simulink model "integrator_12B"  (Simulink 8.0)
settings: Solver=FixedStepDiscrete  StartTime=0.0  StopTime=10.0  FixedStep=1  RelTol=1e-3
libraries: simulink x1
settings Model: Creator=elliocm  LastModifiedBy=elliocm
settings DebuggingCC: IntegerOverflowMsg=none
settings CodeAppCC: CustomSymbolStrType=$N$R$M_T  InternalIdentifier=Shortened
settings ConfigComp: Description=Design Verifier Custom Configuration Component  DVMaxProcessTime=5000  DVMaxTestCaseSteps=500  DVTestSuiteOptimization=CombinedObjectives (Nonlinear Extended)

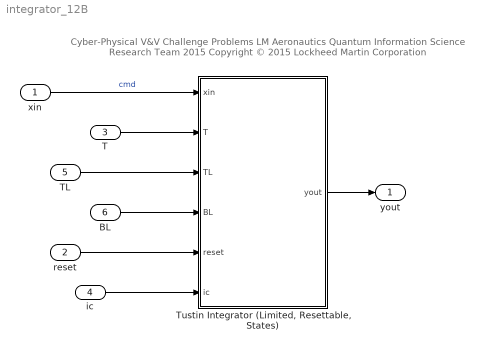
== system integrator_12B ==
  note: Cyber-Physical V&V Challenge Problems
      | LM Aeronautics Quantum Information Science Research Team 2015
      | Copyright © 2015 Lockheed Martin Corporation
  xin : Inport  OutDataTypeStr=double
  reset : Inport  Port=2  OutDataTypeStr=boolean
  T : Inport  Port=3  OutDataTypeStr=double
  ic : Inport  Port=4  OutDataTypeStr=double
  TL : Inport  Port=5  OutDataTypeStr=double
  BL : Inport  Port=6  OutDataTypeStr=double
  "Tustin Integrator (Limited, Resettable, States)" : Subsystem
  yout : Outport
  wires:
  BL/1 -> "Tustin Integrator (Limited, Resettable, States)"/4(BL)
  TL/1 -> "Tustin Integrator (Limited, Resettable, States)"/3(TL)
  reset/1 -> "Tustin Integrator (Limited, Resettable, States)"/5(reset)
  ic/1 -> "Tustin Integrator (Limited, Resettable, States)"/6(ic)
  "Tustin Integrator (Limited, Resettable, States)"/1(yout) -> yout/1
  T/1 -> "Tustin Integrator (Limited, Resettable, States)"/2(T)
  xin/1 -> "Tustin Integrator (Limited, Resettable, States)"/1(xin)  "cmd"

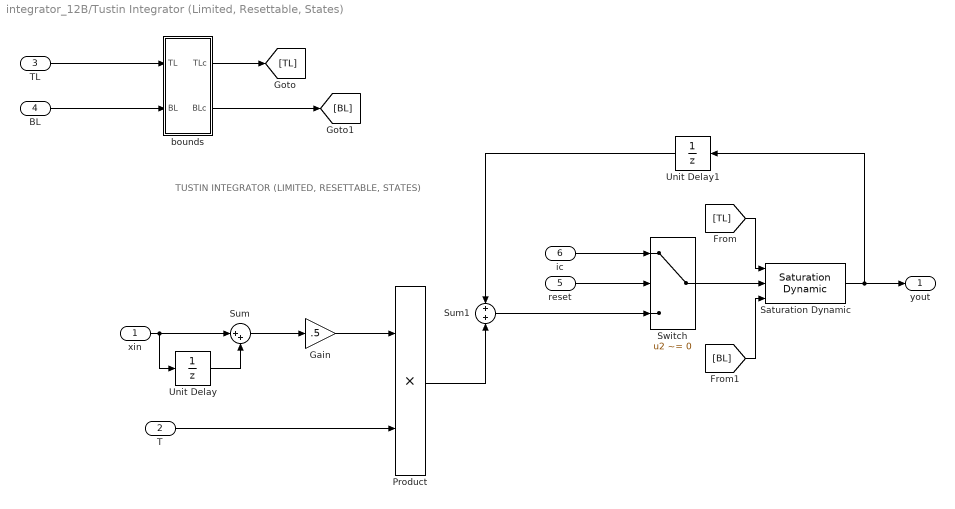
== system integrator_12B/Tustin Integrator (Limited, Resettable, States) ==
  note: TUSTIN INTEGRATOR (LIMITED, RESETTABLE, STATES)
  xin : Inport
  T : Inport  Port=2
  TL : Inport  Port=3
  BL : Inport  Port=4
  reset : Inport  Port=5
  ic : Inport  Port=6
  Gain : Gain  Gain=.5
  Product : Product  RndMeth=Zero
  Saturation Dynamic : simulink/Discontinuities/Saturation Dynamic  OutMin=[]  OutMax=[]  OutDataTypeStr=Inherit: Same as second input  OutDataType=fixdt(1, 16)  OutScaling=2^-10  DoSatur=off
  Sum : Sum  Inputs=|++
  Sum1 : Sum
  Switch : Switch  Criteria=u2 ~= 0  Threshold=0.5
  Unit Delay : UnitDelay  SampleTime=-1
  Unit Delay1 : UnitDelay  SampleTime=-1
  bounds : Subsystem
  yout : Outport
  wires:
  xin/1 -> Unit Delay/1, Sum/1
  Unit Delay/1 -> Sum/2
  Sum/1 -> Gain/1
  Gain/1 -> Product/1
  T/1 -> Product/2
  Product/1 -> Sum1/2
  Sum1/1 -> Switch/3
  reset/1 -> Switch/2
  ic/1 -> Switch/1
  Switch/1 -> Saturation Dynamic/2
  Saturation Dynamic/1 -> Unit Delay1/1, yout/1
  Unit Delay1/1 -> Sum1/1
  TL/1 -> bounds/1(TL)
  BL/1 -> bounds/2(BL)
  bounds/1(TLc) -> [TL]
  bounds/2(BLc) -> [BL]
  [TL] -> Saturation Dynamic/1
  [BL] -> Saturation Dynamic/3

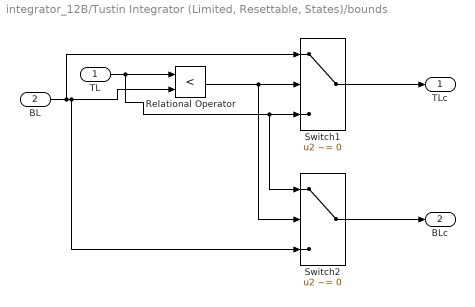
== system integrator_12B/Tustin Integrator (Limited, Resettable, States)/bounds ==
  TL : Inport
  BL : Inport  Port=2
  Relational Operator : RelationalOperator  Operator=<  OutDataTypeStr=boolean
  Switch1 : Switch  Criteria=u2 ~= 0  Threshold=0.5
  Switch2 : Switch  Criteria=u2 ~= 0  Threshold=0.5
  TLc : Outport
  BLc : Outport  Port=2
  wires:
  BL/1 -> Switch1/1, Switch2/3, Relational Operator/2
  TL/1 -> Switch2/1, Switch1/3, Relational Operator/1
  Relational Operator/1 -> Switch2/2, Switch1/2
  Switch1/1 -> TLc/1
  Switch2/1 -> BLc/1
